simulink model "RLC3part2"  (R2018a)
settings: Solver=VariableStepAuto  StartTime=0.0  StopTime=2.0  RelTol=1e-3
libraries: simulink x1
settings Model: Creator=praty  LastModifiedBy=menonpr7
settings DebuggingCC: LibraryContextMissingDiagnostic=warning
settings SFSimCC: SimUseLocalCustomCode=on
settings RTWCC: RTWUseLocalCustomCode=on

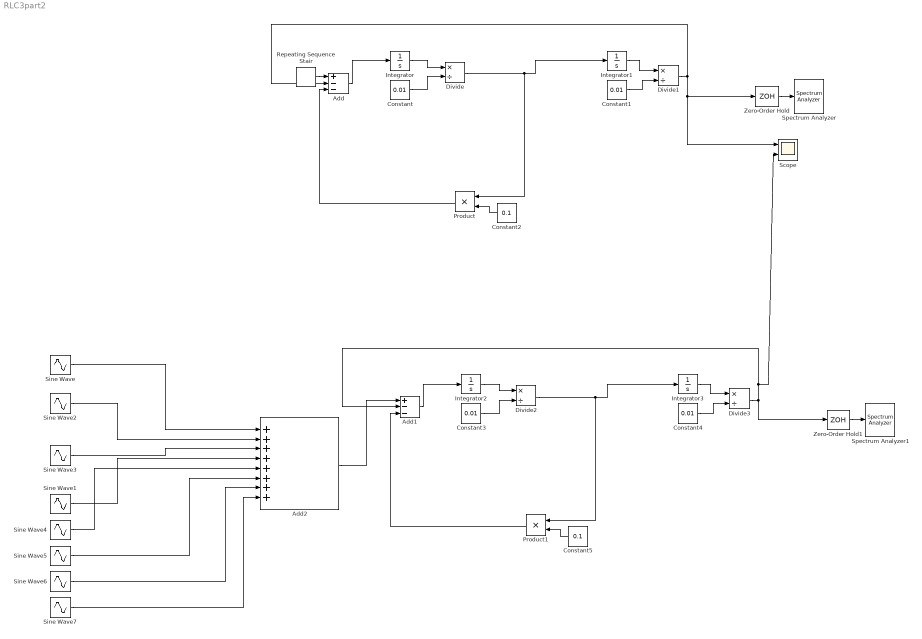
== system RLC3part2 ==
  Add : Sum  Inputs=+--
  Add1 : Sum  Inputs=+--
  Add2 : Sum  Inputs=++++++++
  Constant{,1,3..4} (4 alike) : Constant  Value=0.01
  Constant2 : Constant  Value=0.1
  Constant5 : Constant  Value=0.1
  Divide{,1..3} (4 alike) : Product  Inputs=*/
  Integrator{,1..3} (4 alike) : Integrator
  Product : Product
  Product1 : Product
  Repeating Sequence Stair : simulink/Sources/Repeating Sequence Stair  OutValues=[1 -1]  tsamp=1/64  OutMin=[]  OutMax=[]  OutDataTypeStr=double  OutputDataTypeScalingMode=double  OutDataType=fixdt(0,8)  ConRadixGroup=Best Precision: Vector-wise  OutScaling=2^-12
  Scope : Scope  NumInputPorts=2
  Sine Wave : Sin  Amplitude=4/(7*pi)  Frequency=14*32*pi  SampleTime=0
  Sine Wave1 : Sin  Amplitude=4/pi  Frequency=64*pi  SampleTime=0
  Sine Wave2 : Sin  Amplitude=4/(5*pi)  Frequency=10*32*pi  SampleTime=0
  Sine Wave3 : Sin  Amplitude=4/(3*pi)  Frequency=192*pi  SampleTime=0
  Sine Wave4 : Sin  Amplitude=4/(9*pi)  Frequency=18*32*pi  SampleTime=0
  Sine Wave5 : Sin  Amplitude=4/(11*pi)  Frequency=22*32*pi  SampleTime=0
  Sine Wave6 : Sin  Amplitude=4/(13*pi)  Frequency=26*32*pi  SampleTime=0
  Sine Wave7 : Sin  Amplitude=4/(15*pi)  Frequency=30*32*pi  SampleTime=0
  Spectrum Analyzer : SpectrumAnalyzer
  Spectrum Analyzer1 : SpectrumAnalyzer
  Zero-Order Hold : ZeroOrderHold  SampleTime=2^(-10)
  Zero-Order Hold1 : ZeroOrderHold  SampleTime=2^(-10)
  wires:
  Zero-Order Hold/1 -> Spectrum Analyzer/1
  Integrator/1 -> Divide/1
  Constant/1 -> Divide/2
  Integrator1/1 -> Divide1/1
  Constant1/1 -> Divide1/2
  Divide/1 -> Product/1, Integrator1/1
  Constant2/1 -> Product/2
  Add/1 -> Integrator/1
  Divide1/1 -> Scope/1, Zero-Order Hold/1, Add/2
  Product/1 -> Add/3
  Zero-Order Hold1/1 -> Spectrum Analyzer1/1
  Divide3/1 -> Zero-Order Hold1/1, Scope/2, Add1/2
  Integrator2/1 -> Divide2/1
  Add1/1 -> Integrator2/1
  Constant3/1 -> Divide2/2
  Integrator3/1 -> Divide3/1
  Product1/1 -> Add1/3
  Constant4/1 -> Divide3/2
  Divide2/1 -> Product1/1, Integrator3/1
  Constant5/1 -> Product1/2
  Repeating Sequence Stair/1 -> Add/1
  Sine Wave/1 -> Add2/1
  Sine Wave6/1 -> Add2/7
  Sine Wave4/1 -> Add2/5
  Sine Wave5/1 -> Add2/6
  Sine Wave1/1 -> Add2/4
  Sine Wave7/1 -> Add2/8
  Sine Wave3/1 -> Add2/3
  Sine Wave2/1 -> Add2/2
  Add2/1 -> Add1/1
